simulink model "es1_sim"  (R2022b)
settings: Solver=VariableStepAuto  StartTime=0.0  StopTime=10.0  RelTol=1e-3
settings Model: Creator=claudio  LastModifiedBy=claudio

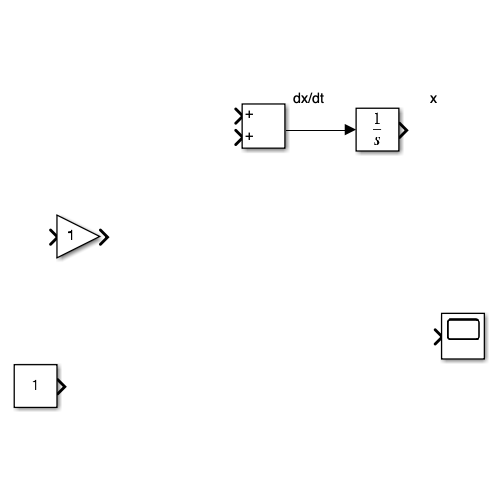
[thumbnail: Simulink's stored preview of the top-level diagram]
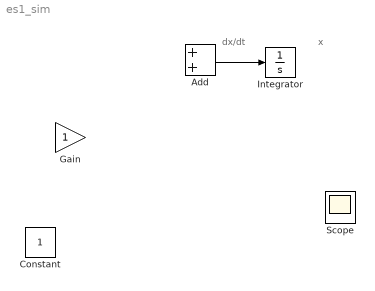
== system es1_sim ==
  note: dx/dt
  note: x
  Add : Sum
  Constant : Constant
  Gain : Gain
  Integrator : Integrator
  Scope : Scope
  wires:
  Add/1 -> Integrator/1
